simulink model "CL_Motor_model_position_control"  (R2020b)
settings: Solver=ode4  StartTime=0.0  StopTime=10.0  FixedStep=.001  RelTol=1e-3
values from neighbouring files (symbols this model uses):
  b = 3.7e-6    (= 3.7e-06)    [position_control.m]    (also in velocity_control.m)
  command = 1    [position_control.m]    (also in velocity_control.m = 12.5663706144)
  J = 8.5e-6    (= 8.5e-06)    [position_control.m]    (also in velocity_control.m)
  K = 0.45    [position_control.m]    (also in velocity_control.m = 0.01591)
  K_a = mean(i_avg ./ V)    [position_control.m]    (also in velocity_control.m)
  K_t = 4.24e-2    (= 0.0424)    [position_control.m]    (also in velocity_control.m)
  p1 = 0.1    [position_control.m]    (also in velocity_control.m = 0)
  p2 = 55    [position_control.m]    (also in velocity_control.m = 70)
  T_friction = 0    [position_control.m]    (also in velocity_control.m = 0.00805)
  T_load = 0    [position_control.m]    (also in velocity_control.m)
  Tau_filter = 0.05    [position_control.m]    (also in velocity_control.m = 0.01)
  time_load = 1    [position_control.m]    (also in velocity_control.m)
  z1 = 0.25    [position_control.m]    (also in velocity_control.m = 0.8)
  z2 = 0.5    [position_control.m]    (also in velocity_control.m = 16.5)
settings Model: Creator=Sangam  LastModifiedBy=aanan
settings DataIOCC: SaveFormat=Array  ReturnWorkspaceOutputs=off
settings DebuggingCC: ArithmeticOperatorsInVariantConditions=warning
settings SFSimCC: CustomCodeUndefinedFunction=UseInterfaceOnly

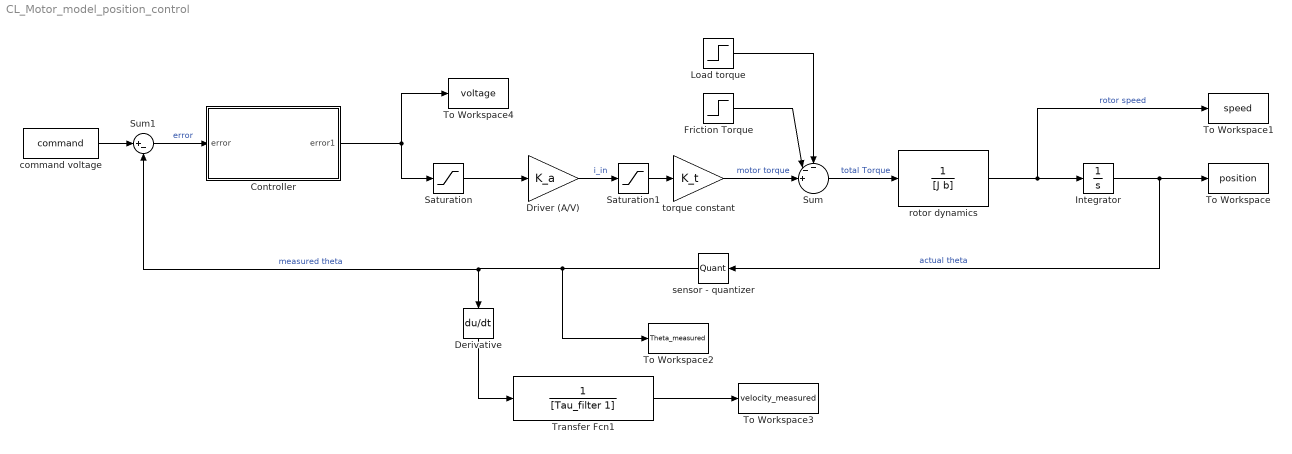
== system CL_Motor_model_position_control ==
  Controller : Subsystem
  Derivative : Derivative
  Driver (A/V) : Gain  Gain=K_a
  Friction Torque : Step  Time=0  After=T_friction  SampleTime=0
  Integrator : Integrator
  Load torque : Step  Time=time_load  After=T_load  SampleTime=0
  Saturation : Saturate  UpperLimit=10  LowerLimit=-10
  Saturation1 : Saturate  UpperLimit=3  LowerLimit=-3
  Sum : Sum  Inputs=--+||
  Sum1 : Sum  Inputs=|+-
  To Workspace : ToWorkspace  VariableName=position  SampleTime=-1
  To Workspace1 : ToWorkspace  VariableName=speed  SampleTime=-1
  To Workspace2 : ToWorkspace  VariableName=Theta_measured  SampleTime=-1
  To Workspace3 : ToWorkspace  VariableName=velocity_measured  SampleTime=-1
  To Workspace4 : ToWorkspace  VariableName=voltage  SampleTime=-1
  Transfer Fcn1 : TransferFcn  Denominator=[Tau_filter 1]
  command voltage : Constant  Value=command
  rotor dynamics : TransferFcn  Denominator=[J b]
  sensor - quantizer : Quantizer  QuantizationInterval=delta_theta
  torque constant : Gain  Gain=K_t
  wires:
  Driver (A/V)/1 -> Saturation1/1  "i_in"
  torque constant/1 -> Sum/3  "motor torque"
  Load torque/1 -> Sum/1
  Friction Torque/1 -> Sum/2
  Sum/1 -> rotor dynamics/1  "total Torque"
  rotor dynamics/1 -> To Workspace1/1, Integrator/1  "rotor speed"
  Integrator/1 -> To Workspace/1, sensor - quantizer/1  "actual theta"
  command voltage/1 -> Sum1/1
  sensor - quantizer/1 -> To Workspace2/1, Sum1/2, Derivative/1  "measured theta"
  Derivative/1 -> Transfer Fcn1/1
  Transfer Fcn1/1 -> To Workspace3/1
  Saturation/1 -> Driver (A/V)/1
  Saturation1/1 -> torque constant/1
  Sum1/1 -> Controller/1(error)  "error"
  Controller/1(error1) -> To Workspace4/1, Saturation/1

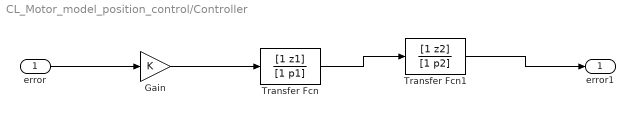
== system CL_Motor_model_position_control/Controller ==
  error : Inport
  Gain : Gain  Gain=K
  Transfer Fcn : TransferFcn  Numerator=[1 z1]  Denominator=[1 p1]
  Transfer Fcn1 : TransferFcn  Numerator=[1 z2]  Denominator=[1 p2]
  error1 : Outport
  wires:
  error/1 -> Gain/1
  Gain/1 -> Transfer Fcn/1
  Transfer Fcn/1 -> Transfer Fcn1/1
  Transfer Fcn1/1 -> error1/1
